simulink model "slo_single_share_pid"  (R2015b)
settings: Solver=FixedStepDiscrete  SolverMode=SingleTasking  StartTime=0.0  StopTime=10  RelTol=1e-3
settings Model: Creator=amatsumo  LastModifiedBy=amatsumo
settings DataIOCC: SaveFormat=Array  SignalLoggingSaveFormat=ModelDataLogs  SaveOutput=off  SignalLogging=off  SaveTime=off
settings OptimizationCC: BlockReduction=off  ConditionallyExecuteInputs=off  DefaultParameterBehavior=Inlined
settings DebuggingCC: AlgebraicLoopMsg=error  UnderspecifiedInitializationDetection=Classic  MergeDetectMultiDrivingBlocksExec=none  SolverPrmCheckMsg=warning  MultiTaskDSMMsg=warning  MultiTaskCondExecSysMsg=none  SingleTaskRateTransMsg=error  StateNameClashWarn=warning
settings HardwareCC: ProdBitPerPointer=32  ProdLargestAtomicFloat=None  ProdIntDivRoundTo=Undefined  ProdEndianess=Unspecified  ProdWordSize=32  ProdHWDeviceType=ASIC/FPGA->ASIC/FPGA  ProdEqTarget=off
settings GRTTargetCC: GeneratePreprocessorConditionals=Disable all
settings ConfigComp: CovModelRefEnable=Off  CovSFcnEnable=off

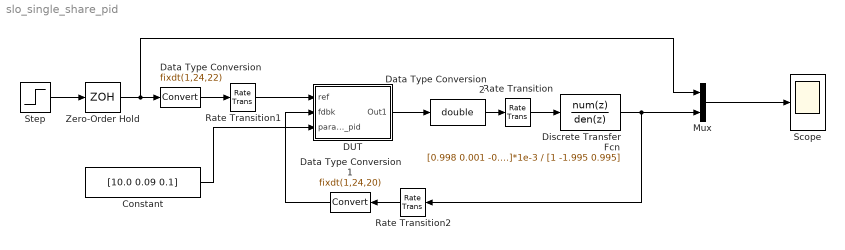
== system slo_single_share_pid ==
  Constant : Constant  Value=[10.0 0.09 0.1]  OutDataTypeStr=fixdt(0,16,11)  SampleTime=-1
  DUT : Subsystem
  Data Type Conversion : DataTypeConversion  OutDataTypeStr=fixdt(1,24,22)  RndMeth=Nearest
  Data Type Conversion1 : DataTypeConversion  OutDataTypeStr=fixdt(1,24,20)  RndMeth=Nearest
  Data Type Conversion2 : DataTypeConversion  OutDataTypeStr=double  RndMeth=Nearest
  Discrete Transfer Fcn : DiscreteTransferFcn  Numerator=[0.998 0.001 -0.997]*1e-3  Denominator=[1 -1.995 0.995]  SampleTime=1/1000
  Mux : Mux  Inputs=2
  Rate Transition : RateTransition  OutPortSampleTime=1/1000
  Rate Transition1 : RateTransition  OutPortSampleTime=1/1000
  Rate Transition2 : RateTransition  OutPortSampleTime=1/1000
  Scope : Scope
  Step : Step  SampleTime=0
  Zero-Order Hold : ZeroOrderHold  SampleTime=1/1000
  wires:
  Step/1 -> Zero-Order Hold/1
  DUT/1(Out1) -> Data Type Conversion2/1
  Discrete Transfer Fcn/1 -> Rate Transition2/1, Mux/2
  Data Type Conversion/1 -> Rate Transition1/1
  Data Type Conversion1/1 -> DUT/2(fdbk)
  Data Type Conversion2/1 -> Rate Transition/1
  Constant/1 -> DUT/3(param_pid)
  Mux/1 -> Scope/1
  Zero-Order Hold/1 -> Mux/1, Data Type Conversion/1
  Rate Transition/1 -> Discrete Transfer Fcn/1
  Rate Transition1/1 -> DUT/1(ref)
  Rate Transition2/1 -> Data Type Conversion1/1

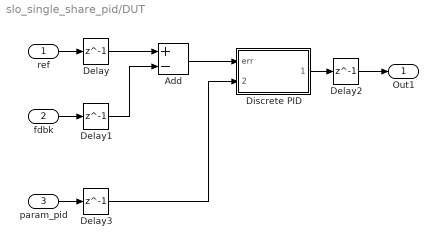
== system slo_single_share_pid/DUT ==
  ref : Inport
  fdbk : Inport  Port=2
  param_pid : Inport  Port=3
  Add : Sum  Inputs=+-  OutDataTypeStr=fixdt(1,24,19)  RndMeth=Nearest
  Delay{,1..3} (4 alike) : Delay  DelayLength=1
  Discrete PID : Subsystem
  Out1 : Outport
  wires:
  fdbk/1 -> Delay1/1
  Discrete PID/1(out_pid) -> Delay2/1
  ref/1 -> Delay/1
  Add/1 -> Discrete PID/1(err)
  Delay/1 -> Add/1
  Delay1/1 -> Add/2
  Delay2/1 -> Out1/1
  param_pid/1 -> Delay3/1
  Delay3/1 -> Discrete PID/2(param_pid)

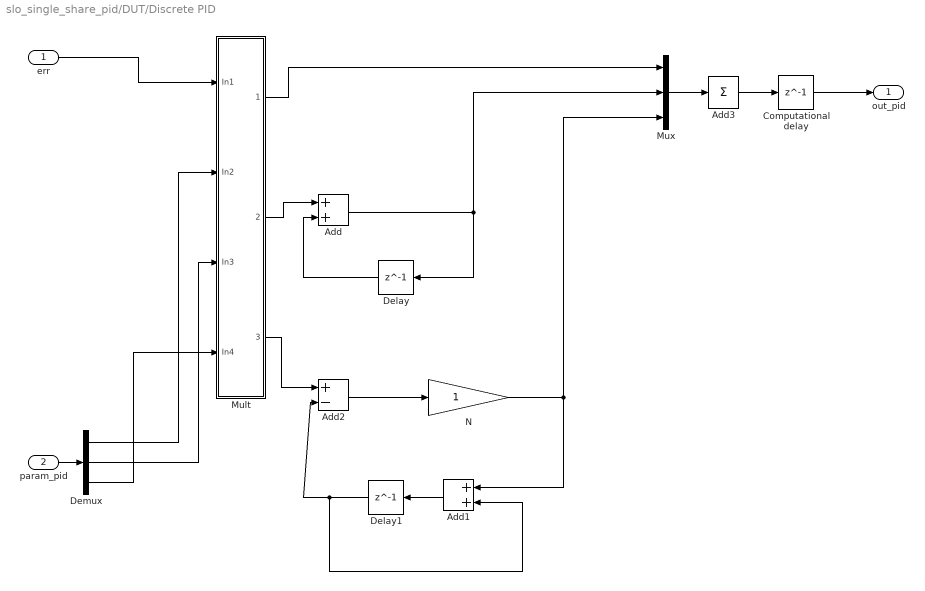
== system slo_single_share_pid/DUT/Discrete PID ==
  err : Inport
  param_pid : Inport  Port=2
  Add : Sum  OutDataTypeStr=Inherit: Same as first input
  Add1 : Sum  OutDataTypeStr=Inherit: Same as first input
  Add2 : Sum  Inputs=+-  OutDataTypeStr=Inherit: Same as first input
  Add3 : Sum  Inputs=+
  Computational delay : Delay  DelayLength=1  InputProcessing=Inherited
  Delay : Delay  DelayLength=1  InputProcessing=Inherited
  Delay1 : Delay  DelayLength=1  InputProcessing=Inherited
  Demux : Demux  Outputs=3
  Mult : Subsystem
      settings: AttributesFormatString=----HDL----\nSharingFactor = 3
  Mux : Mux  Inputs=3
  N : Gain  ParamDataTypeStr=fixdt(0,10,6)  RndMeth=Nearest  OutDataTypeStr=Inherit: Same as input
  out_pid : Outport
  wires:
  Computational delay/1 -> out_pid/1
  Add/1 -> Delay/1, Mux/2
  Delay/1 -> Add/2
  Add1/1 -> Delay1/1
  Delay1/1 -> Add1/2, Add2/2
  Add2/1 -> N/1
  N/1 -> Mux/3, Add1/1
  Add3/1 -> Computational delay/1
  Mux/1 -> Add3/1
  param_pid/1 -> Demux/1
  err/1 -> Mult/1(In1)
  Demux/1 -> Mult/2(In2)
  Demux/2 -> Mult/3(In3)
  Demux/3 -> Mult/4(In4)
  Mult/1(Out1) -> Mux/1
  Mult/2(Out2) -> Add/1
  Mult/3(Out3) -> Add2/1

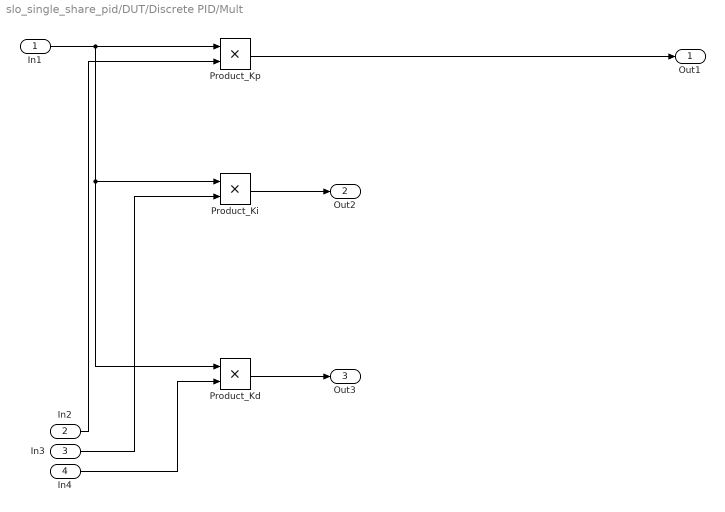
== system slo_single_share_pid/DUT/Discrete PID/Mult ==
  In1 : Inport
  In2 : Inport  Port=2
  In3 : Inport  Port=3
  In4 : Inport  Port=4
  Product_Kd : Product  OutDataTypeStr=fixdt(1,28,23)  RndMeth=Nearest
  Product_Ki : Product  OutDataTypeStr=fixdt(1,28,23)  RndMeth=Nearest
  Product_Kp : Product  OutDataTypeStr=fixdt(1,28,23)  RndMeth=Nearest
  Out1 : Outport
  Out2 : Outport  Port=2
  Out3 : Outport  Port=3
  wires:
  Product_Kp/1 -> Out1/1
  In3/1 -> Product_Ki/2
  In2/1 -> Product_Kp/2
  In4/1 -> Product_Kd/2
  Product_Kd/1 -> Out3/1
  In1/1 -> Product_Kp/1, Product_Kd/1, Product_Ki/1
  Product_Ki/1 -> Out2/1
